simulink model "trab1_questao3_naoLineargrxa"  (R2020a)
settings: Solver=VariableStepAuto  StartTime=0.0  StopTime=10.0  RelTol=1e-3
undefined symbols (not defined in the file or in its folder): sigbuilder_block
settings Model: Creator=luang  LastModifiedBy=luang

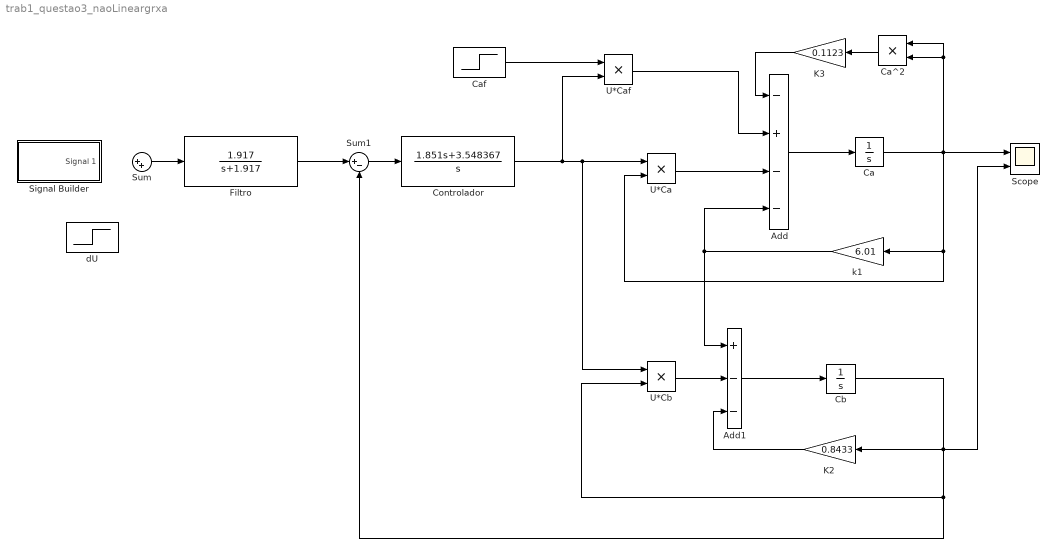
== system trab1_questao3_naoLineargrxa ==
  Add : Sum  Inputs=-+--
  Add1 : Sum  Inputs=+--
  Ca : Integrator
  Ca^2 : Product
  Caf : Step  Time=0  After=5.1  SampleTime=0
  Cb : Integrator
  Controlador : TransferFcn  Numerator=[1.851 3.548367]  Denominator=[1 0]
  Filtro : TransferFcn  Numerator=[1.917]  Denominator=[1 1.917]
  K2 : Gain  Gain=0.8433
  K3 : Gain  Gain=0.1123
  Scope : Scope  NumInputPorts=2
  Signal Builder : Subsystem  Tag=STV Subsys  LoadFcn=sigbuilder_block('load',[437.6 199.2 550.4 400 ]);  StartFcn=sigbuilder_block('start');  StopFcn=sigbuilder_block('stop');  ClipboardFcn=sigbuilder_block('clipboard');  mask(Sigbuilder block){tuvar=[0:10]}
      mask help: Simulink:masks:SigbuilderBlock_MD
      mask init:
      | if ~strcmp(get_param(bdroot(gcbh),'SimulationStatus'),'stopped') tuvar = sigbuilder_block('maskInit'); end
      settings: CopyFcn=sigbuilder_block('copy');  DeleteFcn=sigbuilder_block('delete');  ModelCloseFcn=sigbuilder_block('modelClose');  PreSaveFcn=sigbuilder_block('preSave');  PauseFcn=sigbuilder_block('pause');  ContinueFcn=sigbuilder_block('continue');  NameChangeFcn=sigbuilder_block('namechange');  OpenFcn=sigbuilder_block('open',[437.6 199.2 550.4 400 ]);  CloseFcn=sigbuilder_block('close');
      mask Display: plot(0, 0, 100, 100,[2, 2, 32, 32, 2], [68, 8, 8, 68, 68],[32, 2], [38, 38], [32, 19, 2],[53, 60, 44], [32, 17, 17, 2],[16, 16, 31, 31]);txt = getActiveGroup(gcbh);text(2, 100, txt,'verticalAlignment', 'top');
  Sum : Sum  Inputs=|++
  Sum1 : Sum  Inputs=|+-
  U*Ca : Product
  U*Caf : Product
  U*Cb : Product
  dU : Step  Time=0  After=0.1  SampleTime=0
  k1 : Gain  Gain=6.01
  wires:
  U*Caf/1 -> Add/2
  Caf/1 -> U*Caf/1
  U*Ca/1 -> Add/3
  Add/1 -> Ca/1
  Ca/1 -> Ca^2/2, Ca^2/1, k1/1, U*Ca/2, Scope/1
  Ca^2/1 -> K3/1
  K3/1 -> Add/1
  K2/1 -> Add1/3
  Cb/1 -> U*Cb/2, Sum1/2, Scope/2, K2/1
  U*Cb/1 -> Add1/2
  Add1/1 -> Cb/1
  k1/1 -> Add1/1, Add/4
  Controlador/1 -> U*Cb/1, U*Ca/1, U*Caf/2
  Sum/1 -> Filtro/1
  Filtro/1 -> Sum1/1
  Sum1/1 -> Controlador/1

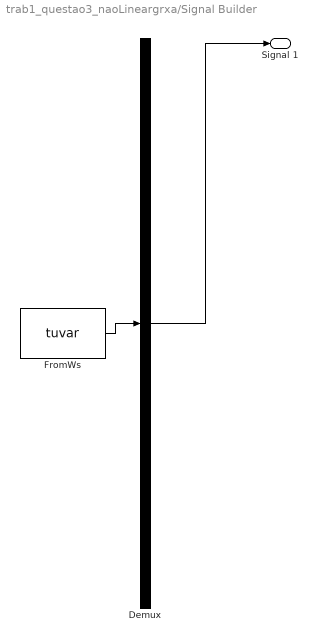
== system trab1_questao3_naoLineargrxa/Signal Builder ==
  Demux : Demux  Tag=STV Demux  Outputs=1
      settings: DisplayOption=none
  FromWs : FromWorkspace  Tag=STV FromWs  VariableName=tuvar
      SigBuilderData=|
      | common.afterFinalStr = 'Extrapolate'
      | common.sampleTime = 0
      | dataSet.timeRange = [0 10]
      | dataSet.name = 'Group 1'
      | sbobj.Groups.Name = 'Group 1'
      | sbobj.Groups.Signals.Name = 'Signal 1'
      | sbobj.Groups.Signals.XData = [0 4 6 6 10]
      | sbobj.Groups.Signals.YData = [0 0 0.995 0 0]
  Signal 1 : Outport  Tag=STV Outport
  wires:
  Demux/1 -> Signal 1/1
  FromWs/1 -> Demux/1
